simulink model "rct_concorde"  (R2020a)
settings: Solver=ode45  StartTime=0.0  StopTime=10  RelTol=1e-3  EnableMultiTasking=on
model workspace (MAT data in the model file):
  G = ss
  G.InputName_ = "\delta_m"
  G.OutputName_ = ["N_z"; "q"]
  G.IOSize_ = [2 1]
  G.Data_ = ltipack.ssdata
  G.Data_.a = [-0.01202  -9.804  -14.88  0  0; 0.0003579  0  0.8524  0  -4.163e-06; -0.0003579  0  -0.8524  1  4.163e-06; 0  0  -2.665  -0.2783  0; 0  234.1  0  0  0]
  G.Data_.b = [0; 0.3113; -0.3113; -4.936; 0]
  G.Data_.c = [0.00853706422018  0  13.5409378186  -0.709225280326  -9.93009174312e-05; 0  0  0  1  0]
  G.Data_.d = [-5.15349643221; 0]
  G.Data_.Delay.Input = 0
  G.Data_.Delay.Output = [0; 0]
  G.Data_.Delay.Internal = []
  G.Data_.Ts = 0
  Kf = 0
  Ki = 0
  Kp = 0
  Kq = 0
  wn = 3
  zeta = 0.8
libraries: cstblocks x1
settings Model: Creator=The MathWorks, Inc.  LastModifiedBy=nikhil
settings DataIOCC: LimitDataPoints=on  SaveFormat=Array  ReturnWorkspaceOutputs=off
settings OptimizationCC: BlockReduction=off  BooleanDataType=off  ExpressionDepthLimit=2147483647  InitFltsAndDblsToZero=on  LifeSpan=inf
settings DebuggingCC: SaveWithParameterizedLinksMsg=none  UnderspecifiedInitializationDetection=Classic  MergeDetectMultiDrivingBlocksExec=none  SignalResolutionControl=TryResolveAllWithWarning  MultiTaskDSMMsg=warning  MultiTaskCondExecSysMsg=none  FcnCallInpInsideContextMsg=warning  StateNameClashWarn=warning  SFUnexpectedBacktrackingDiag=warning  SFNoUnconditionalDefaultTransitionDiag=warning  SFExecutionAtInitializationDiag=none  ArithmeticOperatorsInVariantConditions=warning
settings HardwareCC: ProdBitPerPointer=32  ProdBitPerSizeT=32  ProdBitPerPtrDiffT=32  ProdLargestAtomicFloat=None  ProdIntDivRoundTo=Undefined  ProdEndianess=Unspecified  ProdWordSize=32  ProdHWDeviceType=32-bit Generic  TargetUnknown=on
settings ModelReferenceCC: PropagateSignalLabelsOutOfModel=off
settings SFSimCC: SimUseLocalCustomCode=off  CustomCodeUndefinedFunction=UseInterfaceOnly
settings RTWCC: RTWUseLocalCustomCode=off
settings CodeAppCC: StateflowObjectComments=on
settings GRTTargetCC: TargetFcnLib=ansi_tfl_tmw.mat  TargetLangStandard=C89/C90 (ANSI)  CombineOutputUpdateFcns=off  GRTInterface=on
settings ConfigComp: CovMetricSettings=dw  CovHtmlReporting=on  CovSaveCumulativeToWorkspaceVar=on  CovSaveSingleToWorkspaceVar=on  CovExternalEMLEnable=off  CovSFcnEnable=off

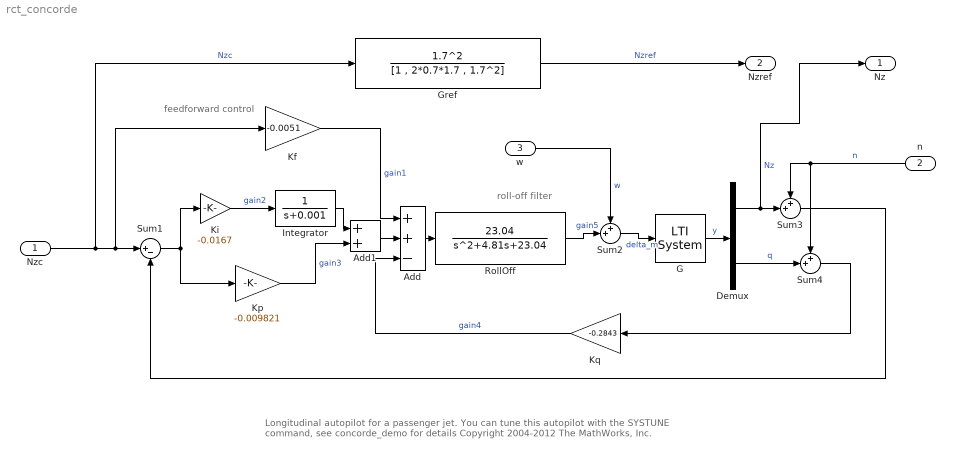
== system rct_concorde ==
  note: feedforward control
  note: roll-off filter
  note: Longitudinal autopilot for a passenger jet.
      |
      | You can tune this autopilot with the SYSTUNE command, see concorde_demo for details
      |
      | Copyright 2004-2012 The MathWorks, Inc.
  Nzc : Inport
  n : Inport  Port=2
  w : Inport  Port=3
  Add : Sum  Inputs=++-
  Add1 : Sum
  Demux : Demux  Outputs=2
      settings: DisplayOption=none
  G : cstblocks/LTI System  sys=G  IC=[]
  Gref : TransferFcn  Numerator=1.7^2  Denominator=[1 , 2*0.7*1.7 , 1.7^2]
  Integrator : TransferFcn  Denominator=[1 0.001]
  Kf : Gain  Gain=-0.0051
  Ki : Gain  Gain=-0.0167
  Kp : Gain  Gain=-0.009821
  Kq : Gain  Gain=-0.2843
  RollOff : TransferFcn  Numerator=[23.04]  Denominator=[1 4.81 23.04]
  Sum1 : Sum  Inputs=|+-  InputSameDT=on  SaturateOnIntegerOverflow=on  OutDataTypeStr=Inherit: Same as first input
  Sum2 : Sum  Inputs=++|
  Sum3 : Sum  Inputs=++|
  Sum4 : Sum  Inputs=++|
  Nz : Outport  VectorParamsAs1DForOutWhenUnconnected=off
  Nzref : Outport  Port=2
  wires:
  G/1 -> Demux/1  "y"
  Nzc/1 -> Gref/1, Sum1/1, Kf/1  "Nzc"
  Demux/2 -> Sum4/2  "q"
  Add/1 -> RollOff/1
  Sum1/1 -> Kp/1, Ki/1
  Ki/1 -> Integrator/1  "gain2"
  Kp/1 -> Add1/2  "gain3"
  Kq/1 -> Add/3  "gain4"
  Add1/1 -> Add/2
  Kf/1 -> Add/1  "gain1"
  Gref/1 -> Nzref/1  "Nzref"
  n/1 -> Sum4/1, Sum3/1  "n"
  Sum3/1 -> Sum1/2
  Sum4/1 -> Kq/1
  RollOff/1 -> Sum2/2  "gain5"
  Sum2/1 -> G/1  "delta_m"
  w/1 -> Sum2/1  "w"
  Integrator/1 -> Add1/1
  Demux/1 -> Nz/1, Sum3/2  "Nz"
